simulink model "PositionControl"  (Simulink 8.2)
settings: Solver=FixedStepDiscrete  StartTime=0.0  StopTime=Inf  RelTol=1e-3
PreLoadFcn:
  | Ts=0.001;
libraries: speedgoatlib_IO102 x3, speedgoatlib_IO301 x3, xpclib x2, xpcutilitieslib x1, simulink x1
settings Model: Creator=LukePH  LastModifiedBy=LukePH  SimulationMode=external  BufferReuse=off
settings DataIOCC: SignalLoggingSaveFormat=Dataset
settings OptimizationCC: BlockReduction=off  OptimizeBlockIOStorage=off  BufferReuse=off  ExpressionFolding=off  ExpressionDepthLimit=128  LocalBlockOutputs=off
settings DebuggingCC: FcnCallInpInsideContextMsg=EnableAllAsError  StateNameClashWarn=none
settings HardwareCC: ProdIntDivRoundTo=Zero  ProdEndianess=LittleEndian  ProdHWDeviceType=Generic->32-bit x86 compatible
settings RTWCC: SystemTargetFile=xpctarget.tlc  TemplateMakefile=xpc_default_tmf  Description=xPC Target  ProcessScript=xpctarget_make_rtw_hook  RTWCompilerOptimization=On
settings xpcTargetCC: TargetFcnLib=ansi_tfl_table_tmw.mat  CodeReplacementLibrary=XPC_BLAS  ParMdlRefBuildCompliant=on  ConcurrentExecutionCompliant=on  CombineSignalStateStructs=off  MATLABClassNameForMDSCustomization=xpcAperiodicCustomization  GRTInterface=on  GenerateAllocFcn=off  xPCTaskExecutionProfile=off  xPCRL32EventNumber=5000  xPCLoadParamSetFile=off  xPCConcurrentTasks=off  xPCEnableSFAnimation=off

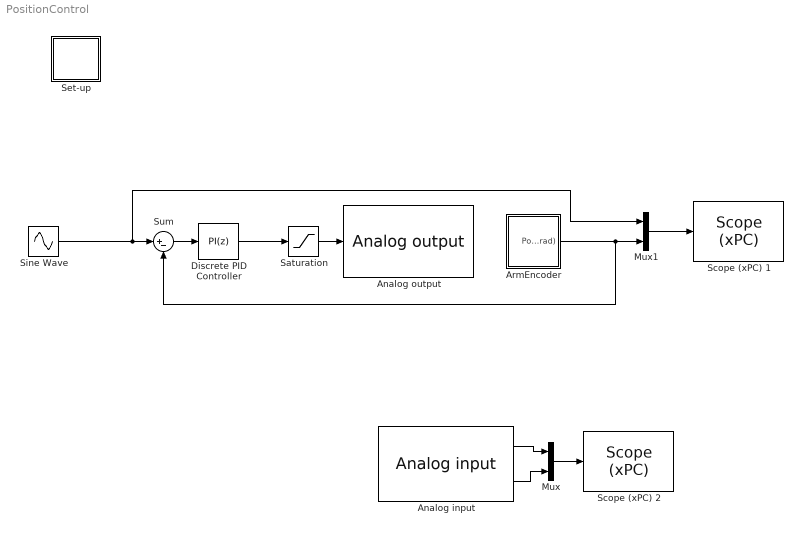
== system PositionControl ==
  Analog input : speedgoatlib_IO102/Analog input  id=1  channels=[1,2]  range=1  high_voltage=off  adCoupling=2  ts=Ts  pciSlot=-1
  Analog output : speedgoatlib_IO102/Analog output  id=1  channels=1  range=1  ts=Ts  pciSlot=-1
  ArmEncoder : Subsystem
  Discrete PID Controller : simulink/Continuous/PID Controller  Controller=PI  TimeDomain=Discrete-time  SampleTime=Ts  IntegratorMethod=Forward Euler  FilterMethod=Forward Euler  Form=Parallel  P=50  I=1  D=0  N=100  InitialConditionSource=internal  InitialConditionForIntegrator=0  InitialConditionForFilter=0  ExternalReset=none  LimitOutput=on  UpperSaturationLimit=5  LowerSaturationLimit=-5  LinearizeAsGain=off  AntiWindupMode=clamping  Kb=1  TrackingMode=off  Kt=1  PParamMin=[]  PParamMax=[]  IParamMin=[]  IParamMax=[]  DParamMin=[]  DParamMax=[]  NParamMin=[]  NParamMax=[]  KbParamMin=[]  KbParamMax=[]  KtParamMin=[]  KtParamMax=[]  POutMin=[]  POutMax=[]  IOutMin=[]  IOutMax=[]  DOutMin=[]  DOutMax=[]  NOutMin=[]  NOutMax=[]  KbOutMin=[]  KbOutMax=[]  KtOutMin=[]  KtOutMax=[]  IntegratorOutMin=[]  IntegratorOutMax=[]  FilterOutMin=[]  FilterOutMax=[]  SumOutMin=[]  SumOutMax=[]  SumI1OutMin=[]  SumI1OutMax=[]  SumI2OutMin=[]  SumI2OutMax=[]  SumI3OutMin=[]  SumI3OutMax=[]  SumDOutMin=[]  SumDOutMax=[]  SaturationOutMin=[]  SaturationOutMax=[]  IntegratorContinuousStateAttributes=''  IntegratorStateMustResolveToSignalObject=off  IntegratorRTWStateStorageClass=Auto  FilterContinuousStateAttributes=''  FilterStateMustResolveToSignalObject=off  FilterRTWStateStorageClass=Auto
  Mux : Mux  Inputs=2
  Mux1 : Mux  Inputs=2
  Saturation : Saturate  UpperLimit=5  LowerLimit=-5
  Scope (xPC) 1 : xpclib/Misc./Scope (xPC)   scopeno=1  scopetype=Target  autostart=on  viewmode=Graphical redraw  formatstr='%15.6f'  grid=on  ylimits=[-2*pi,2*pi]  nosamples=250  noprepostsamples=0  interleave=1  triggermode=FreeRun  triggersignal=1  trigsignalfromport=off  triggerlevel=0.0  triggerslope=Either  triggerscope=1  triggersample=0  filename=data.dat  mode=Lazy  writesize=512  autorestart=off  dynamicfilemode=off  maxwritefilesize=512*1024^2
  Scope (xPC) 2 : xpclib/Misc./Scope (xPC)   scopeno=2  scopetype=Target  autostart=on  viewmode=Graphical redraw  formatstr='%15.6f'  grid=on  ylimits=[-5,5]  nosamples=250  noprepostsamples=0  interleave=1  triggermode=FreeRun  triggersignal=1  trigsignalfromport=off  triggerlevel=0.0  triggerslope=Either  triggerscope=1  triggersample=0  filename=data.dat  mode=Lazy  writesize=512  autorestart=off  dynamicfilemode=off  maxwritefilesize=512*1024^2
  Set-up : Subsystem
  Sine Wave : Sin  Amplitude=pi/4  Bias=pi  SampleTime=0
  Sum : Sum  Inputs=|+-
  wires:
  Analog input/2 -> Mux/2
  Mux/1 -> Scope (xPC) 2/1
  ArmEncoder/1(Pos (rad)) -> Sum/2, Mux1/2
  Analog input/1 -> Mux/1
  Sum/1 -> Discrete PID Controller/1
  Discrete PID Controller/1 -> Saturation/1
  Saturation/1 -> Analog output/1
  Mux1/1 -> Scope (xPC) 1/1
  Sine Wave/1 -> Mux1/1, Sum/1

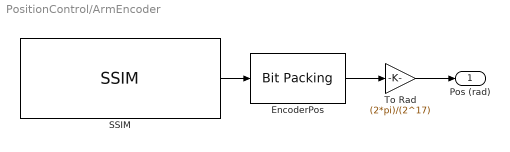
== system PositionControl/ArmEncoder ==
  EncoderPos : xpcutilitieslib/Bit Packing   MaskBitPatterns={[0:16]}  MaskPackDataType=int32  MaskPackDataSize=[1]
  SSIM : speedgoatlib_IO301/SSI/SSIM  id=1  chan=[1]  coding=Gray  clockDivider=[200]  wordSize=[17]  TL=[0]  TP=[990]  ssiminv=off  ts=Ts  pciSlot=-1
  To Rad : Gain  Gain=(2*pi)/(2^17)  OutDataTypeStr=double
  Pos (rad) : Outport
  wires:
  SSIM/1 -> EncoderPos/1
  EncoderPos/1 -> To Rad/1
  To Rad/1 -> Pos (rad)/1

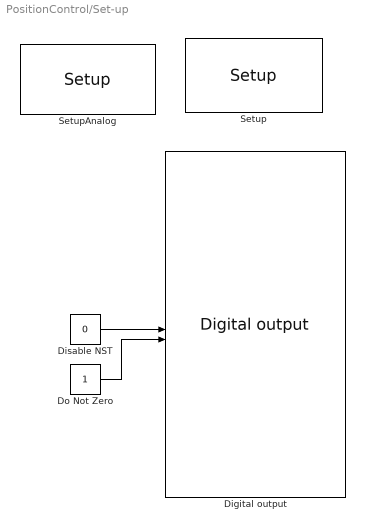
== system PositionControl/Set-up ==
  Digital output : speedgoatlib_IO301/DIO/Digital output  id=1  channelGroup=Lower  portType=32 ports of type double  lowerDirection=[0,0,0,0,0,0,1,1,1,1,1,1,1,1,1,1]  upperDirection=[1,1,1,1,1,1,1,1,0,0,0,0,0,0,0,0]  ts=Ts  pciSlot=-1
  Disable NST : Constant  Value=0
  Do Not Zero : Constant
  Setup : speedgoatlib_IO301/Setup/Setup  group=Module setup  id=1  fpga1=speedgoat_IO301_CI_01230  pciSlot=-1  lowerDirection=[0,0,0,0,0,0,1,1,1,1,1,1,1,1,1,1]  lowerReset=[1]  lowerValue=[1]  upperDirection=[1, 1, 1, 1, 1, 1, 1, 1, 0, 0, 0, 0, 0, 0, 0, 0]  upperReset=[1]  upperValue=[0]
  SetupAnalog : speedgoatlib_IO102/Setup  group=Module setup  id=1  range=+-10V  cal=off  pciSlot=-1  adChannelMode=Multiple-channel (enter number of channels below)  adChannel=2  adCoupling=Single-ended  daChannel=[1]  daReset=[1]  daInitValue=[0]  diChannel=[1]  doChannel=[1]  doReset=[1]  doInitValue=[0]
  wires:
  Disable NST/1 -> Digital output/17
  Do Not Zero/1 -> Digital output/18
